simulink model "watering"  (R2018b)
settings: Solver=VariableStepAuto  StartTime=0.0  StopTime=intervals  RelTol=1e-3
libraries: simulink x1
settings Model: Creator=Filipowicz_user1  LastModifiedBy=jf

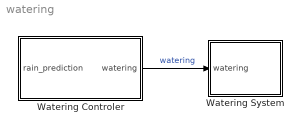
== system watering ==
  Watering Controler : Subsystem
  Watering System : Subsystem
  wires:
  Watering Controler/1(watering) -> Watering System/1(watering)  "watering"

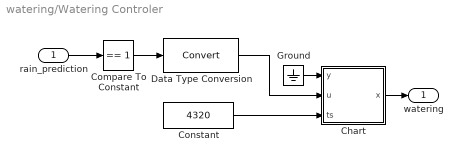
== system watering/Watering Controler ==
  rain_prediction : Inport
  Chart : Stateflow chart  TreatAsAtomicUnit=on
  Compare To Constant : simulink/Logic and Bit Operations/Compare To Constant  relop===  const=1  OutDataTypeStr=boolean
  Constant : Constant  Value=4320
  Data Type Conversion : DataTypeConversion
  Ground : Ground
  watering : Outport
  wires:
  Chart/1(x) -> watering/1
  Constant/1 -> Chart/3(ts)
  rain_prediction/1 -> Compare To Constant/1
  Compare To Constant/1 -> Data Type Conversion/1
  Data Type Conversion/1 -> Chart/2(u)
  Ground/1 -> Chart/1(y)

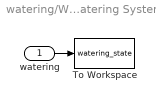
== system watering/Watering System ==
  watering : Inport
  To Workspace : ToWorkspace  VariableName=watering_state  SaveFormat=Timeseries  SampleTime=-1
  wires:
  watering/1 -> To Workspace/1

== stateflow chart watering/Watering Controler/Chart ==
  settings: updateMethod=DISCRETE  sampleTime=1  executeAtInitialization=1
  state Idle
    x=0;
    t1=ts/timeStep;
  state State1
    x=1;
  state Wait
  (default) -> Idle
  Idle -> Idle [order 2]
  Wait -> Idle [order 2] : after(t1,'sec')
  Idle -> State1 [order 1] : [u>=1]
  State1 -> Idle [order 2] : [y==1]
  State1 -> Wait [order 1] : [u==0]
  Wait -> State1 [order 1] : [u==1]
  data: y input; u input; x output; ts input; timeStep constant double; t1 local
